simulink model "task2_2_2"  (R2020a)
settings: Solver=FixedStepAuto  StartTime=0.0  StopTime=60  FixedStep=0.01  RelTol=1e-3
settings Model: Creator=dell  LastModifiedBy=dell

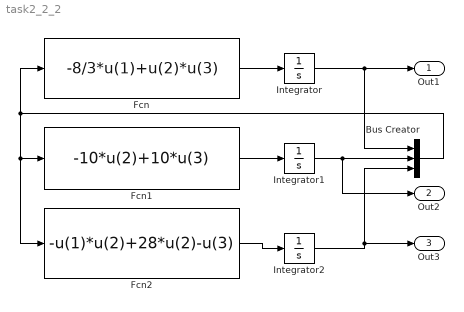
== system task2_2_2 ==
  Bus Creator : BusCreator  Inputs=3
  Fcn : Fcn  Expr=-8/3*u(1)+u(2)*u(3)
  Fcn1 : Fcn  Expr=-10*u(2)+10*u(3)
  Fcn2 : Fcn  Expr=-u(1)*u(2)+28*u(2)-u(3)
  Integrator : Integrator
  Integrator1 : Integrator
  Integrator2 : Integrator  InitialCondition=0.001
  Out1 : Outport
  Out2 : Outport  Port=2
  Out3 : Outport  Port=3
  wires:
  Bus Creator/1 -> Fcn2/1, Fcn1/1, Fcn/1
  Fcn/1 -> Integrator/1
  Fcn1/1 -> Integrator1/1
  Fcn2/1 -> Integrator2/1
  Integrator/1 -> Out1/1, Bus Creator/1
  Integrator2/1 -> Out3/1, Bus Creator/3
  Integrator1/1 -> Out2/1, Bus Creator/2
